simulink model "effector"  (R2025a)
settings: Solver=ode45  StartTime=0.0  StopTime=200  RelTol=1e-3
values from neighbouring files (symbols this model uses):
  A = [ ... (first row only)    [effector_setup.m]
  B = [ ... (first row only)    [effector_setup.m]
  C = eye(4)    [effector_setup.m]
  D = zeros(4, 2)    [effector_setup.m]
  Initial = zeros(4, 1)    [effector_setup.m]
libraries: spsStairGeneratorLib x1
settings Model: Creator=rajap  LastModifiedBy=rajap

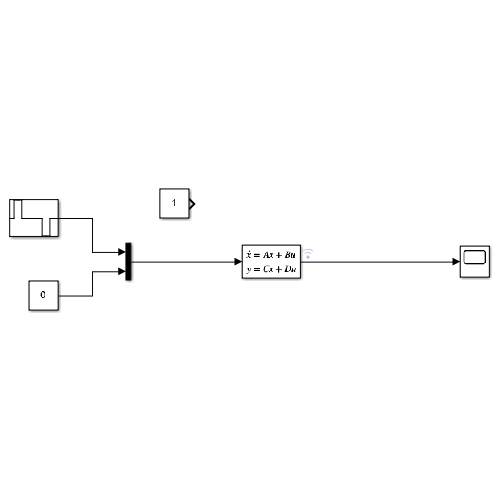
[thumbnail: Simulink's stored preview of the top-level diagram]
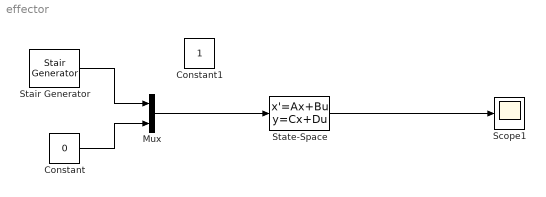
== system effector ==
  Constant : Constant  Value=0
  Constant1 : Constant
  Mux : Mux  Inputs=2
  Scope1 : Scope
      settings: ActiveDisplayYMinimum=-9.5810698525022886  ActiveDisplayYMaximum=44.940227411570049
  Stair Generator : spsStairGeneratorLib/Stair Generator  t=[0, 1, 2, 3, 4, 5, 6, 7, 8, 9, 10, 11, 12, 13]  e=[0, 0, 0.1, 0.1, 0, 0, 0, 0, 0, -0.1, -0.1, 0, 0, 0]  Ts=0
  State-Space : StateSpace  A=A  B=B  C=C  D=D  InitialCondition=Initial
  wires:
  Constant/1 -> Mux/2
  Mux/1 -> State-Space/1
  State-Space/1 -> Scope1/1
  Stair Generator/1 -> Mux/1
